simulink model "ufss_full"  (R2022b)
settings: Solver=VariableStepAuto  StartTime=0.0  StopTime=70  RelTol=1e-3
InitFcn:
  | K1 = 1;
  | K2 = 1;
settings Model: Creator=Zonularity  LastModifiedBy=Zonularity

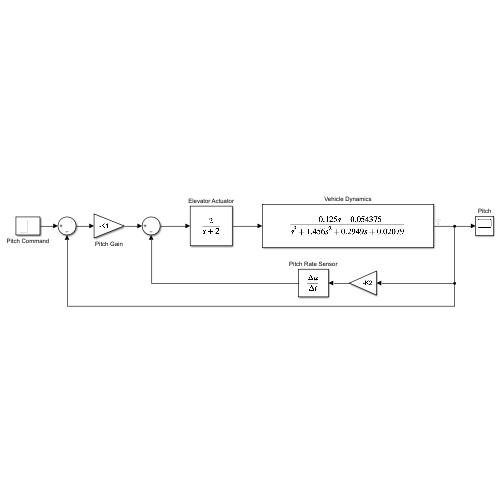
[thumbnail: Simulink's stored preview of the top-level diagram]
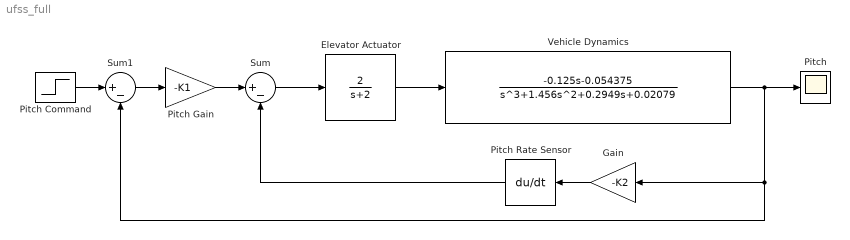
== system ufss_full ==
  Elevator Actuator : TransferFcn  Numerator=[2]  Denominator=[1 2]
  Gain : Gain  Gain=-K2
  Pitch : Scope
  Pitch Command : Step  SampleTime=0
  Pitch Gain : Gain  Gain=-K1
  Pitch Rate Sensor : Derivative
  Sum : Sum  Inputs=|+-
  Sum1 : Sum  Inputs=|+-
  Vehicle Dynamics : TransferFcn  Numerator=[0, 0, -0.125, -0.054375]  Denominator=[1, 1.456, 0.2949, 0.02079]
  wires:
  Gain/1 -> Pitch Rate Sensor/1
  Pitch Rate Sensor/1 -> Sum/2
  Sum/1 -> Elevator Actuator/1
  Elevator Actuator/1 -> Vehicle Dynamics/1
  Pitch Gain/1 -> Sum/1
  Sum1/1 -> Pitch Gain/1
  Vehicle Dynamics/1 -> Pitch/1, Sum1/2, Gain/1
  Pitch Command/1 -> Sum1/1
